simulink model "control_matlab_visualization"  (R2023a)
settings: Solver=FixedStepAuto  StartTime=0.0  StopTime=500  FixedStep=1e-2  RelTol=1e-3
model workspace (MAT data in the model file):
  SL_ROS_VariableLengthArrays_MaxSizes.CommonInfo.ArrayTruncateAction = 'EmitWarning'
  SL_ROS_VariableLengthArrays_MaxSizes.MsgTypeMap = containers.Map
  SL_ROS_VariableLengthArrays_MaxSizes.MsgTypeMap.serialization.keys = {'sgtdv_msgs/Point2DArr'}
  SL_ROS_VariableLengthArrays_MaxSizes.MsgTypeMap.serialization.values{1}.PropertyName = 'Points'
  SL_ROS_VariableLengthArrays_MaxSizes.MsgTypeMap.serialization.values{1}.DataType = 'sgtdv_msgs/Point2D'
  SL_ROS_VariableLengthArrays_MaxSizes.MsgTypeMap.serialization.values{1}.MaxLength = 512
  SL_ROS_VariableLengthArrays_MaxSizes.MsgTypeMap.serialization.uniformity = 0
  SL_ROS_VariableLengthArrays_MaxSizes.MsgTypeMap.serialization.keyType = 'char'
  SL_ROS_VariableLengthArrays_MaxSizes.MsgTypeMap.serialization.valueType = 'any'
libraries: robotlib x6
settings Model: Creator=gugo  LastModifiedBy=gugo
settings OptimizationCC: EnhancedBackFolding=on  PassReuseOutputArgsAs=Individual arguments  ZeroExternalMemoryAtStartup=off  ZeroInternalMemoryAtStartup=off  MaxStackSize=64  OptimizeBlockOrder=speed  DifferentSizesBufferReuse=on  OptimizationCustomize=off  EfficientTunableParamExpr=on
settings DebuggingCC: ParameterTunabilityLossMsg=error
settings HardwareCC: ProdBitPerPointer=32  ProdBitPerSizeT=32  ProdBitPerPtrDiffT=32  ProdLargestAtomicFloat=None  ProdIntDivRoundTo=Undefined  ProdEndianess=Unspecified  ProdWordSize=32  ProdHWDeviceType=Generic->Unspecified (assume 32-bit Generic)  UseEmbeddedCoderFeatures=off
settings SFSimCC: MATLABDynamicMemAlloc=off
settings RTWCC: Description=Embedded Coder  SystemTargetFile=ert.tlc  HardwareBoard=Robot Operating System (ROS)  TLCOptions="-aInlineSetEventsForThisBaseRateFcn=TLC_FALSE -aSuppressMultiTaskScheduler=TLC_FALSE  -aRateBasedStepFcn=0"  TemplateMakefile=ert_default_tmf  Toolchain=Catkin  TargetLang=C++
settings CodeAppCC: ForceParamTrailComments=on  IgnoreCustomStorageClasses=off  OperatorAnnotations=on  SimulinkDataObjDesc=on  SFDataObjDesc=on  InsertBlockDesc=on
settings ERTTargetCC: SupportNonInlinedSFcns=on

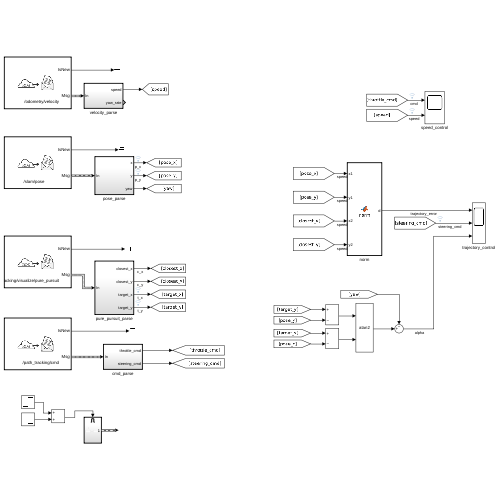
[thumbnail: Simulink's stored preview of the top-level diagram]
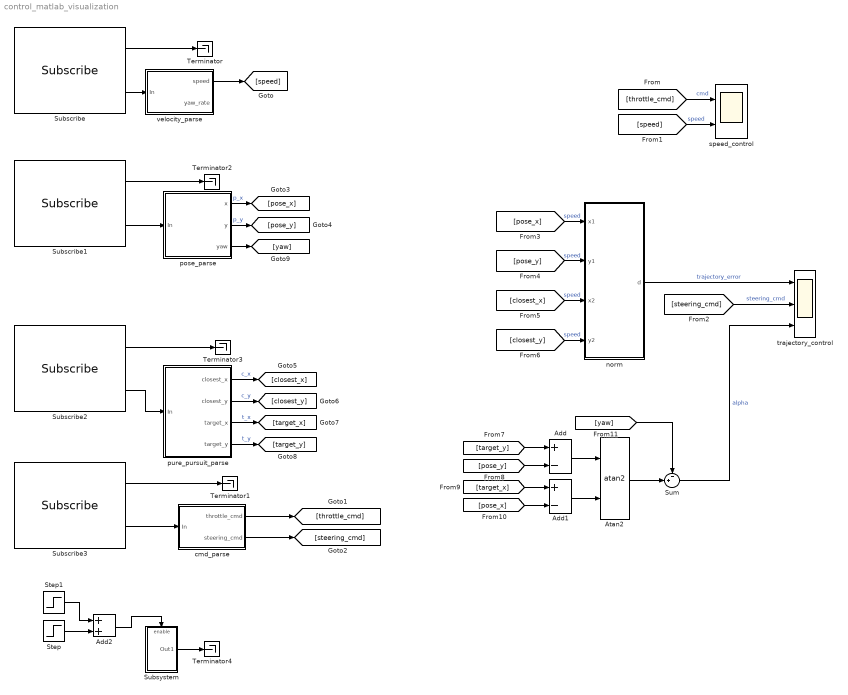
== system control_matlab_visualization ==
  Add : Sum  Inputs=+-
  Add1 : Sum  Inputs=+-
  Add2 : Sum
  Atan2 : Trigonometry  Operator=atan2
  Step : Step  Time=1.01  After=-1  SampleTime=0
  Step1 : Step  SampleTime=0
  Subscribe : robotlib/Subscribe  topicSource=Select from ROS network  topic=/odometry/velocity  messageType=sgtdv_msgs/CarVel  SampleTime=-1  legacyBusStruct=off  messageQueueLength=1
  Subscribe1 : robotlib/Subscribe  topicSource=Select from ROS network  topic=/slam/pose  messageType=sgtdv_msgs/CarPose  SampleTime=-1  legacyBusStruct=off  messageQueueLength=1
  Subscribe2 : robotlib/Subscribe  topicSource=Select from ROS network  topic=/path_tracking/visualize/pure_pursuit  messageType=visualization_msgs/MarkerArray  SampleTime=-1  legacyBusStruct=off  messageQueueLength=1
  Subscribe3 : robotlib/Subscribe  topicSource=Select from ROS network  topic=/path_tracking/cmd  messageType=sgtdv_msgs/Control  SampleTime=-1  legacyBusStruct=off  messageQueueLength=1
  Subsystem : Subsystem
  Sum : Sum  Inputs=-+|
  Terminator{,1..4} (5 alike) : Terminator
  cmd_parse : Subsystem  TreatAsAtomicUnit=on
  norm : MATLAB Function  TreatAsAtomicUnit=on
  pose_parse : Subsystem  TreatAsAtomicUnit=on
  pure_pursuit_parse : Subsystem  TreatAsAtomicUnit=on
  speed_control : Scope  NumInputPorts=2
  trajectory_control : Scope  NumInputPorts=3
  velocity_parse : Subsystem  TreatAsAtomicUnit=on
  wires:
  Subscribe/1 -> Terminator/1
  Subscribe/2 -> velocity_parse/1(In)
  Subscribe1/2 -> pose_parse/1(In)
  Subscribe1/1 -> Terminator2/1
  Subscribe2/1 -> Terminator3/1
  Subscribe2/2 -> pure_pursuit_parse/1(In)
  Subscribe3/2 -> cmd_parse/1(In)
  Subscribe3/1 -> Terminator1/1
  velocity_parse/1(speed) -> [speed]
  cmd_parse/1(throttle_cmd) -> [throttle_cmd]
  cmd_parse/2(steering_cmd) -> [steering_cmd]
  [throttle_cmd] -> speed_control/1  "cmd"
  [speed] -> speed_control/2  "speed"
  pose_parse/1(x) -> [pose_x]  "p_x"
  pose_parse/2(y) -> [pose_y]  "p_y"
  pure_pursuit_parse/1(closest_x) -> [closest_x]  "c_x"
  pure_pursuit_parse/2(closest_y) -> [closest_y]  "c_y"
  [pose_x] -> norm/1(x1)  "speed"
  [pose_y] -> norm/2(y1)  "speed"
  [closest_x] -> norm/3(x2)  "speed"
  [closest_y] -> norm/4(y2)  "speed"
  norm/1(d) -> trajectory_control/1  "trajectory_error"
  pure_pursuit_parse/3(target_x) -> [target_x]  "t_x"
  pure_pursuit_parse/4(target_y) -> [target_y]  "t_y"
  [target_y] -> Add/1
  [pose_y] -> Add/2
  [pose_x] -> Add1/2
  [target_x] -> Add1/1
  Add/1 -> Atan2/1
  Add1/1 -> Atan2/2
  Atan2/1 -> Sum/2
  pose_parse/3(yaw) -> [yaw]
  [yaw] -> Sum/1
  Sum/1 -> trajectory_control/3  "alpha"
  [steering_cmd] -> trajectory_control/2  "steering_cmd"
  Step/1 -> Add2/2
  Step1/1 -> Add2/1
  Add2/1 -> Subsystem/Enable
  Subsystem/1(Out1) -> Terminator4/1

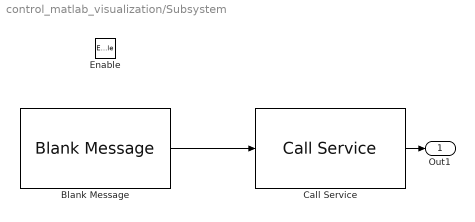
== system control_matlab_visualization/Subsystem ==
  Enable : EnablePort
  Blank Message : robotlib/Blank Message  messageClass=Service Request  entityType=std_srvs/Empty  messageType=std_srvs/EmptyRequest  SampleTime=inf  legacyBusStruct=off
  Call Service : robotlib/Call Service  topicSource=Select from ROS network  service=/path_tracking/start  serviceType=std_srvs/Empty  connectionTimeout=5  keepPersistent=off  ShowErrorCodeOutput=off  legacyBusStruct=off
  Out1 : Outport
  wires:
  Blank Message/1 -> Call Service/1
  Call Service/1 -> Out1/1

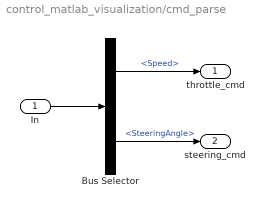
== system control_matlab_visualization/cmd_parse ==
  In : Inport
  Bus Selector : BusSelector  OutputSignals=Speed,SteeringAngle
  throttle_cmd : Outport
  steering_cmd : Outport  Port=2
  wires:
  Bus Selector/1 -> throttle_cmd/1  "<Speed>"
  In/1 -> Bus Selector/1
  Bus Selector/2 -> steering_cmd/1  "<SteeringAngle>"

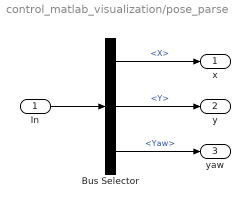
== system control_matlab_visualization/pose_parse ==
  In : Inport
  Bus Selector : BusSelector  OutputSignals=Position.X,Position.Y,Yaw
  x : Outport
  y : Outport  Port=2
  yaw : Outport  Port=3
  wires:
  Bus Selector/2 -> y/1  "<Y>"
  Bus Selector/1 -> x/1  "<X>"
  In/1 -> Bus Selector/1
  Bus Selector/3 -> yaw/1  "<Yaw>"

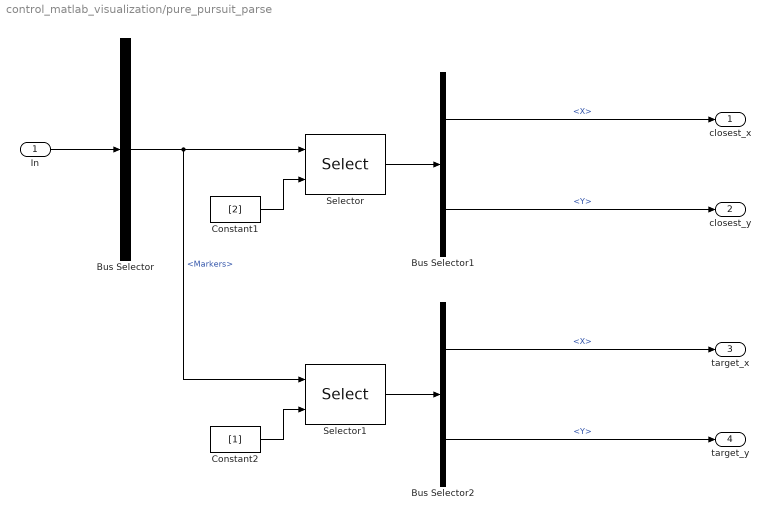
== system control_matlab_visualization/pure_pursuit_parse ==
  In : Inport
  Bus Selector : BusSelector  OutputSignals=Markers
  Bus Selector1 : BusSelector  OutputSignals=Pose.Position.X,Pose.Position.Y
  Bus Selector2 : BusSelector  OutputSignals=Pose.Position.X,Pose.Position.Y
  Constant1 : Constant  Value=[2]
  Constant2 : Constant  Value=[1]
  Selector : Selector  IndexOptions=Index vector (port)  Indices=[2]  OutputSizes=1
  Selector1 : Selector  IndexOptions=Index vector (port)  Indices=[2]  OutputSizes=1
  closest_x : Outport
  closest_y : Outport  Port=2
  target_x : Outport  Port=3
  target_y : Outport  Port=4
  wires:
  In/1 -> Bus Selector/1
  Bus Selector/1 -> Selector1/1, Selector/1  "<Markers>"
  Bus Selector1/2 -> closest_y/1  "<Y>"
  Bus Selector1/1 -> closest_x/1  "<X>"
  Constant1/1 -> Selector/2
  Selector/1 -> Bus Selector1/1
  Selector1/1 -> Bus Selector2/1
  Constant2/1 -> Selector1/2
  Bus Selector2/1 -> target_x/1  "<X>"
  Bus Selector2/2 -> target_y/1  "<Y>"

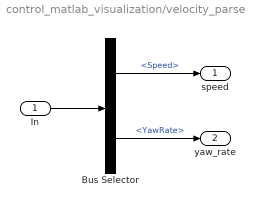
== system control_matlab_visualization/velocity_parse ==
  In : Inport
  Bus Selector : BusSelector  OutputSignals=Speed,YawRate
  speed : Outport
  yaw_rate : Outport  Port=2
  wires:
  In/1 -> Bus Selector/1
  Bus Selector/1 -> speed/1  "<Speed>"
  Bus Selector/2 -> yaw_rate/1  "<YawRate>"

== matlab function control_matlab_visualization/norm ==
  data: x1 input; d output; y1 input; x2 input; y2 input
function d = norm(x1, y1, x2, y2)

d = norm([x1; y1] - [x2; y2]);
